simulink model "RC_Tiefpass_Gleichspannung"  (R2022a)
settings: Solver=VariableStepAuto  StartTime=0.0  StopTime=1  RelTol=1e-6
undefined symbols (not defined in the file): C, R, ue_hat
settings Model: Creator=Gianluca  LastModifiedBy=Gianluca

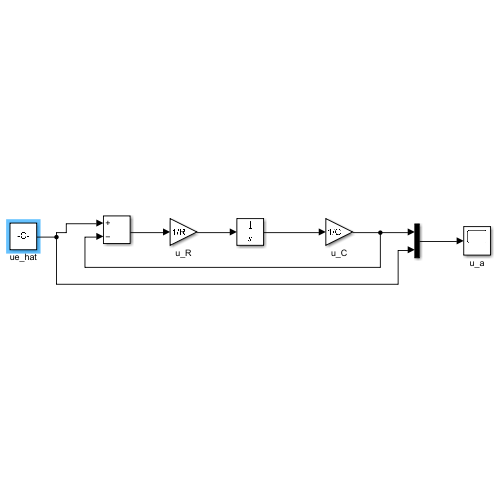
[thumbnail: Simulink's stored preview of the top-level diagram]
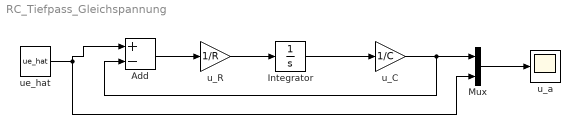
== system RC_Tiefpass_Gleichspannung ==
  Add : Sum  Inputs=+-
  Integrator : Integrator
  Mux : Mux  Inputs=2
  u_C : Gain  Gain=1/C
  u_R : Gain  Gain=1/R
  u_a : Scope
  ue_hat : Constant  Value=ue_hat
  wires:
  u_C/1 -> Add/2, Mux/1
  Integrator/1 -> u_C/1
  ue_hat/1 -> Add/1, Mux/2
  u_R/1 -> Integrator/1
  Add/1 -> u_R/1
  Mux/1 -> u_a/1
